simulink model "ecuacion_tiempo"  (R2022b)
settings: Solver=VariableStepAuto  StartTime=0.0  StopTime=10.0  RelTol=1e-3
settings Model: Creator=Nacho Andrade  LastModifiedBy=Nacho Andrade

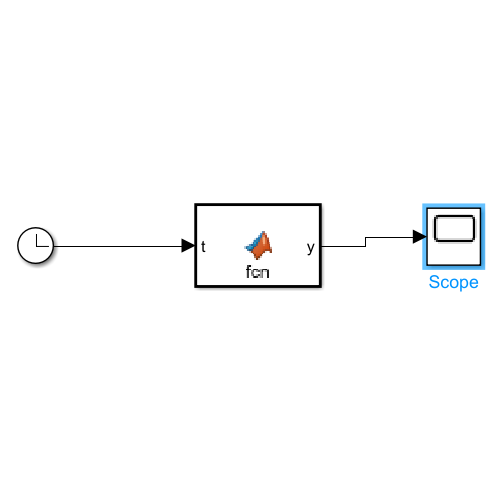
[thumbnail: Simulink's stored preview of the top-level diagram]
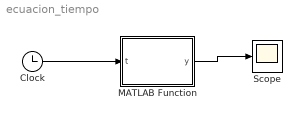
== system ecuacion_tiempo ==
  Clock : Clock
  MATLAB Function : MATLAB Function  TreatAsAtomicUnit=on
  Scope : Scope
  wires:
  Clock/1 -> MATLAB Function/1(t)
  MATLAB Function/1(y) -> Scope/1

== matlab function ecuacion_tiempo/MATLAB Function ==
  data: t input; y output
function y = fcn(t)

y = 1-(exp(-7*t).*cos(sqrt(51).*t))-((7/sqrt(51)).*exp(-7*t).*sin(sqrt(51).*t));
